simulink model "singleTank_2016a"  (R2016a)
settings: Solver=ode4  SolverMode=SingleTasking  StartTime=0.0  StopTime=1000  FixedStep=0.5  RelTol=1e-3
settings Model: Creator=ngoan  LastModifiedBy=ngoan
settings DataIOCC: ReturnWorkspaceOutputs=on
settings DebuggingCC: UnconnectedInputMsg=none  UnconnectedOutputMsg=none  UnconnectedLineMsg=none  SFUnexpectedBacktrackingDiag=error  SFNoUnconditionalDefaultTransitionDiag=error
settings SFSimCC: SimUseLocalCustomCode=on
settings RTWCC: RTWUseLocalCustomCode=on
settings GRTTargetCC: TargetLangStandard=C99 (ISO)
settings ConfigComp: CovMetricSettings=dwe  CovSaveCumulativeToWorkspaceVar=off  CovSaveSingleToWorkspaceVar=off  CovExternalEMLEnable=on

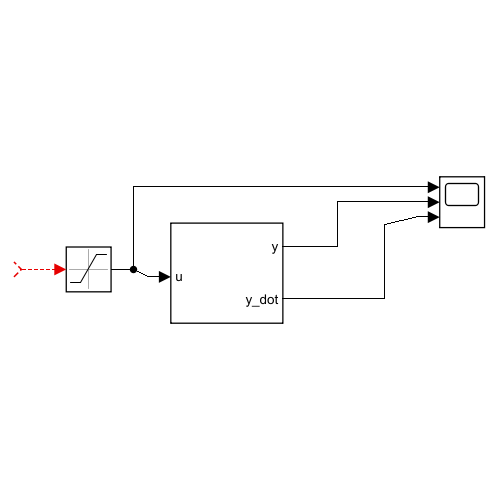
[thumbnail: Simulink's stored preview of the top-level diagram]
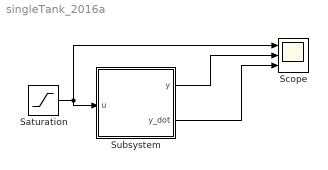
== system singleTank_2016a ==
  Saturation : Saturate  UpperLimit=12  LowerLimit=0
  Scope : Scope  NumInputPorts=3
  Subsystem : Subsystem
  wires:
  Subsystem/2(y_dot) -> Scope/3
  ? -> Saturation/1
  Subsystem/1(y) -> Scope/2
  Saturation/1 -> Scope/1, Subsystem/1(u)

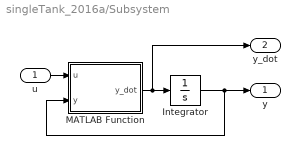
== system singleTank_2016a/Subsystem ==
  u : Inport
  Integrator : Integrator
  MATLAB Function : MATLAB Function  TreatAsAtomicUnit=on
  y : Outport
  y_dot : Outport  Port=2
  wires:
  MATLAB Function/1(y_dot) -> y_dot/1, Integrator/1
  Integrator/1 -> y/1, MATLAB Function/2(y)
  u/1 -> MATLAB Function/1(u)

== matlab function singleTank_2016a/Subsystem/MATLAB Function ==
  data: u input; y_dot output; y input
function y_dot = fcn(u,y)
K = 140 ; % HE so may bom (cm^3/s/V)
C = 0.9 ; % He so nhot
g = 981; % gia toc trong truong (cm/s^2)
A = 314 ; % Tiet dien bon nuoc (cm^2)
y_dot = (K*u - C*sqrt(2*g*y))/A;
